simulink model "PID_PD_gesamt"  (R2016b)
settings: Solver=VariableStepAuto  StartTime=0.0  StopTime=60  RelTol=1e-3
settings Model: Creator=Fritz  LastModifiedBy=Fritz

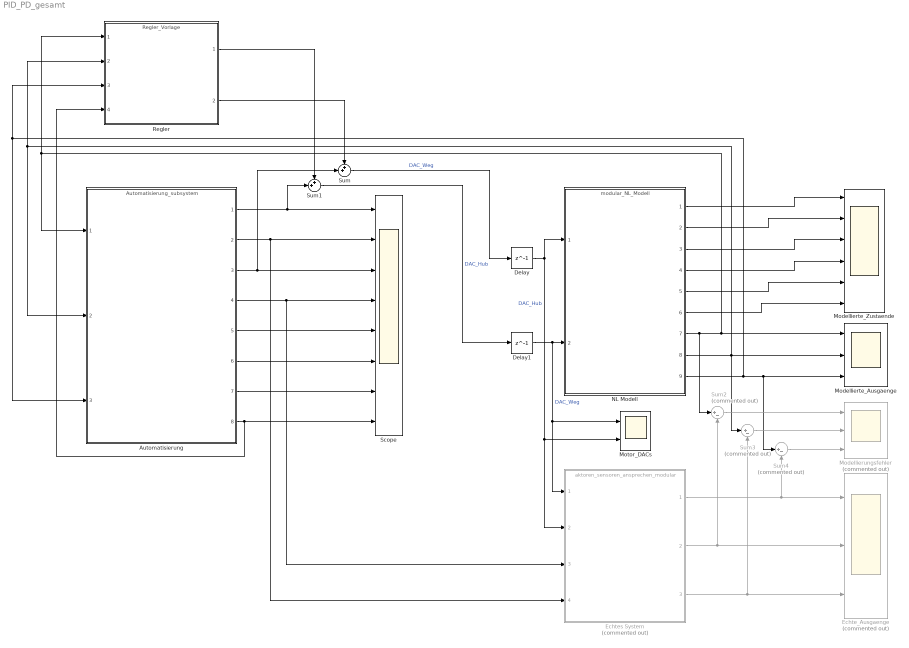
== system PID_PD_gesamt ==
  Automatisierung : ModelReference  ModelNameDialog=Automatisierung_subsystem.slx  SimulationMode=Normal  ModelReferenceVersion=1.73
  Delay : Delay  DelayLength=1
  Delay1 : Delay  DelayLength=1
  Echte_Ausgaenge : Scope  Commented=on  NumInputPorts=3
  Echtes System : ModelReference  Commented=on  ModelNameDialog=aktoren_sensoren_ansprechen_modular.slx  SimulationMode=Normal  ModelReferenceVersion=1.21
  Modellierte_Ausgaenge : Scope  NumInputPorts=3
  Modellierte_Zustaende : Scope  NumInputPorts=6
  Modellierungsfehler : Scope  Commented=on  NumInputPorts=3
  Motor_DACs : Scope  NumInputPorts=2
  NL Modell : ModelReference  ModelNameDialog=modular_NL_Modell.slx  SimulationMode=Normal  ModelReferenceVersion=1.4
  Regler : ModelReference  ModelNameDialog=Regler_Vorlage.slx  SimulationMode=Normal  ModelReferenceVersion=1.3
  Scope : Scope  NumInputPorts=8
  Sum : Sum  Inputs=++|
  Sum1 : Sum  Inputs=++|
  Sum2 : Sum  Commented=on  Inputs=|+-
  Sum3 : Sum  Commented=on  Inputs=|+-
  Sum4 : Sum  Commented=on  Inputs=|+-
  wires:
  NL Modell/1 -> Modellierte_Zustaende/1
  NL Modell/2 -> Modellierte_Zustaende/2
  NL Modell/3 -> Modellierte_Zustaende/3
  NL Modell/4 -> Modellierte_Zustaende/4
  NL Modell/5 -> Modellierte_Zustaende/5
  NL Modell/6 -> Modellierte_Zustaende/6
  NL Modell/7 -> Modellierte_Ausgaenge/1, Regler/1, Automatisierung/1, Sum2/1
  NL Modell/8 -> Sum3/1, Modellierte_Ausgaenge/2, Regler/2, Automatisierung/2
  NL Modell/9 -> Sum4/1, Modellierte_Ausgaenge/3, Regler/3, Automatisierung/3
  Echtes System/1 -> Sum4/2, Echte_Ausgaenge/1
  Echtes System/2 -> Echte_Ausgaenge/2, Sum2/2
  Echtes System/3 -> Sum3/2, Echte_Ausgaenge/3
  Sum/1 -> Delay/1  "DAC_Weg"
  Sum1/1 -> Delay1/1  "DAC_Hub"
  Automatisierung/1 -> Scope/1, Sum1/2
  Automatisierung/3 -> Scope/3, Sum/2
  Regler/2 -> Sum/1
  Regler/1 -> Sum1/1
  Sum2/1 -> Modellierungsfehler/1
  Sum3/1 -> Modellierungsfehler/2
  Sum4/1 -> Modellierungsfehler/3
  Delay1/1 -> Motor_DACs/1, Echtes System/1, NL Modell/2  "DAC_Weg"
  Delay/1 -> NL Modell/1, Motor_DACs/2, Echtes System/2  "DAC_Hub"
  Automatisierung/8 -> Scope/8, Regler/4
  Automatisierung/2 -> Scope/2, Echtes System/4
  Automatisierung/4 -> Scope/4, Echtes System/3
  Automatisierung/5 -> Scope/5
  Automatisierung/6 -> Scope/6
  Automatisierung/7 -> Scope/7
